simulink model "Grading"  (R2021b)
settings: Solver=FixedStepDiscrete  StartTime=0.0  StopTime=10.0  RelTol=1e-3  EnableMultiTasking=on
settings Model: Creator=fady  LastModifiedBy=fady
settings DataIOCC: ReturnWorkspaceOutputs=off
settings OptimizationCC: DefaultParameterBehavior=Inlined  InlineInvariantSignals=on  EnableMemcpy=off  LifeSpan=1  EfficientTunableParamExpr=on
settings DebuggingCC: UnderspecifiedInitializationDetection=Classic  MergeDetectMultiDrivingBlocksExec=none  SFMachineParentedDataDiag=warning  ArithmeticOperatorsInVariantConditions=warning
settings ModelReferenceCC: PropagateSignalLabelsOutOfModel=off
settings SFSimCC: MATLABDynamicMemAlloc=off  CustomCodeUndefinedFunction=UseInterfaceOnly
settings RTWCC: Description=Embedded Coder  SystemTargetFile=ert.tlc  GenCodeOnly=on  TemplateMakefile=ert_default_tmf  GenerateReport=on  IncludeHyperlinkInReport=on  LaunchReport=on  GenerateTraceInfo=on  GenerateTraceReport=on  GenerateTraceReportSl=on  GenerateTraceReportSf=on  GenerateTraceReportEml=on
settings CodeAppCC: ForceParamTrailComments=on  IgnoreCustomStorageClasses=off  OperatorAnnotations=on  SimulinkDataObjDesc=on  SFDataObjDesc=on  MATLABFcnDesc=on  InsertBlockDesc=on  StateflowObjectComments=on  MATLABSourceComments=on
settings ERTTargetCC: MultiwordLength=2048  GenerateSampleERTMain=on  InlinedParameterPlacement=NonHierarchical  ERTCustomFileTemplate=example_file_process.tlc

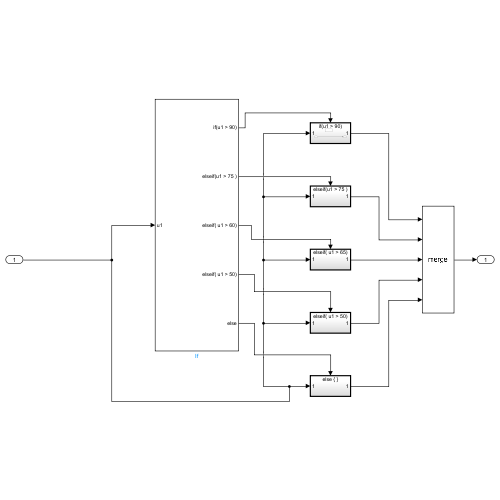
[thumbnail: Simulink's stored preview of the top-level diagram]
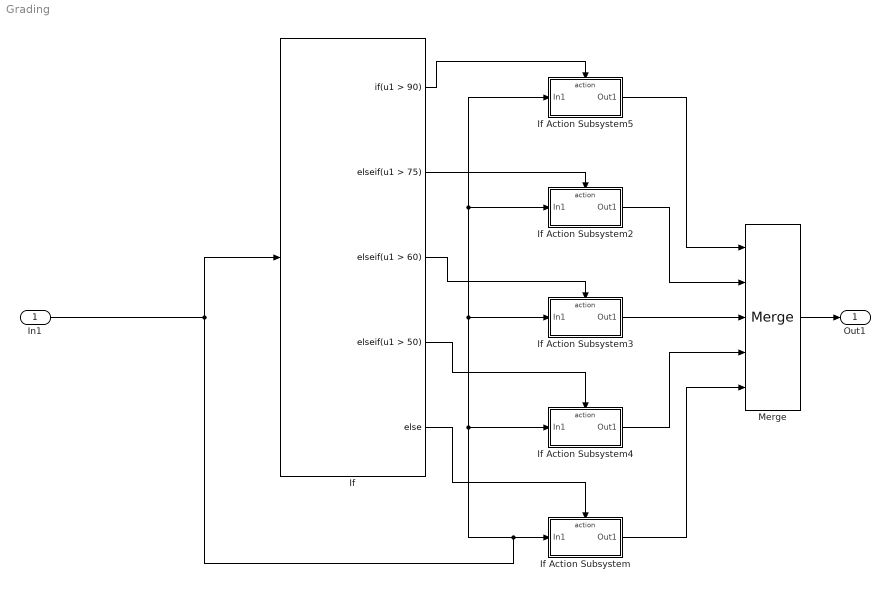
== system Grading ==
  In1 : Inport  OutDataTypeStr=uint8
  If : If  IfExpression=u1 > 90  ElseIfExpressions=u1 > 75 , u1 > 60, u1 > 50
  If Action Subsystem : Subsystem  TreatAsAtomicUnit=on
  If Action Subsystem2 : Subsystem  TreatAsAtomicUnit=on
  If Action Subsystem3 : Subsystem  TreatAsAtomicUnit=on
  If Action Subsystem4 : Subsystem  TreatAsAtomicUnit=on
  If Action Subsystem5 : Subsystem  TreatAsAtomicUnit=on
  Merge : Merge  Inputs=5
  Out1 : Outport
  wires:
  If/2 -> If Action Subsystem2/Action
  In1/1 -> If/1, If Action Subsystem2/1(In1), If Action Subsystem5/1(In1), If Action Subsystem3/1(In1), If Action Subsystem4/1(In1), If Action Subsystem/1(In1)
  If Action Subsystem4/1(Out1) -> Merge/4
  If/3 -> If Action Subsystem3/Action
  If Action Subsystem2/1(Out1) -> Merge/2
  Merge/1 -> Out1/1
  If Action Subsystem/1(Out1) -> Merge/5
  If/4 -> If Action Subsystem4/Action
  If Action Subsystem3/1(Out1) -> Merge/3
  If Action Subsystem5/1(Out1) -> Merge/1
  If/1 -> If Action Subsystem5/Action
  If/5 -> If Action Subsystem/Action

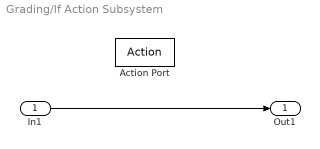
== system Grading/If Action Subsystem ==
  In1 : Inport
  Action Port : ActionPort  ActionPortLabel=else
  Out1 : Outport
  wires:
  In1/1 -> Out1/1

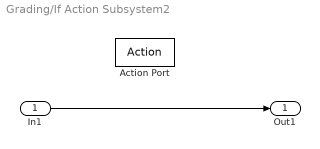
== system Grading/If Action Subsystem2 ==
  In1 : Inport
  Action Port : ActionPort  ActionPortLabel=elseif(u1 > 75 )
  Out1 : Outport
  wires:
  In1/1 -> Out1/1

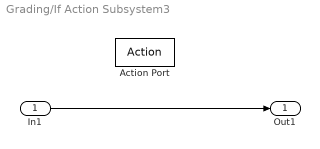
== system Grading/If Action Subsystem3 ==
  In1 : Inport
  Action Port : ActionPort  ActionPortLabel=elseif( u1 > 60)
  Out1 : Outport
  wires:
  In1/1 -> Out1/1

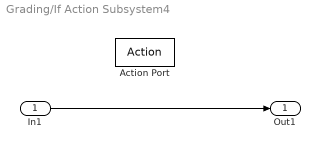
== system Grading/If Action Subsystem4 ==
  In1 : Inport
  Action Port : ActionPort  ActionPortLabel=elseif( u1 > 50)
  Out1 : Outport
  wires:
  In1/1 -> Out1/1

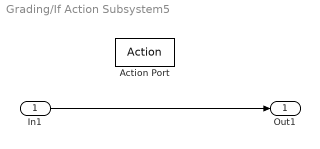
== system Grading/If Action Subsystem5 ==
  In1 : Inport
  Action Port : ActionPort  ActionPortLabel=if(u1 > 90)
  Out1 : Outport
  wires:
  In1/1 -> Out1/1
